simulink model "model_regulator"  (R2018a)
settings: Solver=ode45  StartTime=0.0  StopTime=500  RelTol=1e-3  EnableMultiTasking=on
values from neighbouring files (symbols this model uses):
  A = ans.A    [main.m]
  B = ans.B    [main.m]
  g1 = g(1)    [main.m]
  g2 = g(2)    [main.m]
  q11 = Q(1,1)    [main.m]
  q22 = Q(2,2)    [main.m]
  R = backup.R    [main.m]
undefined symbols (not defined in the file or in its folder): magnitude
libraries: simulink x3
settings Model: Creator=Vlad2  LastModifiedBy=Admin
settings DataIOCC: LimitDataPoints=on  SaveFormat=Array
settings OptimizationCC: LifeSpan=inf
settings DebuggingCC: SolverPrmCheckMsg=warning  SFUnexpectedBacktrackingDiag=warning  SFNoUnconditionalDefaultTransitionDiag=warning  SFExecutionAtInitializationDiag=none
settings HardwareCC: ProdBitPerPointer=32  ProdBitPerSizeT=32  ProdBitPerPtrDiffT=32  ProdLargestAtomicFloat=None  ProdIntDivRoundTo=Undefined  ProdEndianess=Unspecified  ProdWordSize=32  ProdHWDeviceType=32-bit Generic
settings ModelReferenceCC: PropagateSignalLabelsOutOfModel=off
settings CodeAppCC: StateflowObjectComments=on
settings GRTTargetCC: TargetLangStandard=C89/C90 (ANSI)  GeneratePreprocessorConditionals=Disable all
settings ConfigComp: CovMetricSettings=dw  CovHtmlReporting=on  CovSaveCumulativeToWorkspaceVar=on  CovSaveSingleToWorkspaceVar=on  CovExternalEMLEnable=off  CovSFcnEnable=off

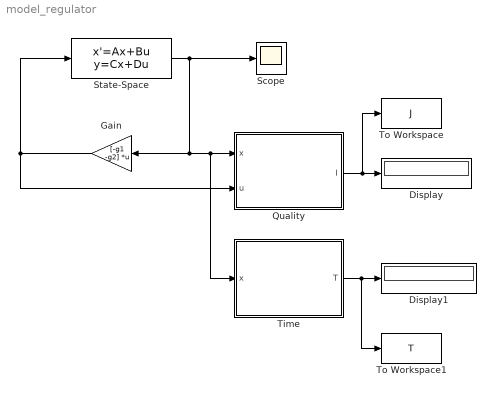
== system model_regulator ==
  Display : Display
  Display1 : Display
  Gain : Gain  Gain=[-g1 -g2]  Multiplication=Matrix(K*u)
  Quality : Subsystem
  Scope : Scope
  State-Space : StateSpace  A=A  B=B  C=eye(2)  D=[0;0]  InitialCondition=[1;1]
  "Time " : Subsystem
  To Workspace : ToWorkspace  VariableName=J  SaveFormat=Timeseries  SampleTime=-1
  To Workspace1 : ToWorkspace  VariableName=T  SaveFormat=Timeseries  SampleTime=-1
  wires:
  Quality/1(I) -> To Workspace/1, Display/1
  "Time "/1(T) -> To Workspace1/1, Display1/1
  Gain/1 -> Quality/2(u), State-Space/1
  State-Space/1 -> Scope/1, Gain/1, "Time "/1(x), Quality/1(x)

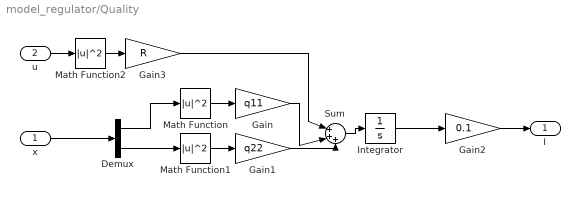
== system model_regulator/Quality ==
  x : Inport
  u : Inport  Port=2
  Demux : Demux  Outputs=2
  Gain : Gain  Gain=q11
  Gain1 : Gain  Gain=q22
  Gain2 : Gain  Gain=0.1
  Gain3 : Gain  Gain=R
  Integrator : Integrator
  Math Function : Math  Operator=magnitude^2  SaturateOnIntegerOverflow=on
  Math Function1 : Math  Operator=magnitude^2  SaturateOnIntegerOverflow=on
  Math Function2 : Math  Operator=magnitude^2  SaturateOnIntegerOverflow=on
  Sum : Sum  Inputs=|+++
  I : Outport
  wires:
  x/1 -> Demux/1
  Demux/1 -> Math Function/1
  Demux/2 -> Math Function1/1
  Math Function/1 -> Gain/1
  Math Function1/1 -> Gain1/1
  Math Function2/1 -> Gain3/1
  u/1 -> Math Function2/1
  Gain3/1 -> Sum/1
  Gain/1 -> Sum/2
  Gain1/1 -> Sum/3
  Sum/1 -> Integrator/1
  Integrator/1 -> Gain2/1
  Gain2/1 -> I/1

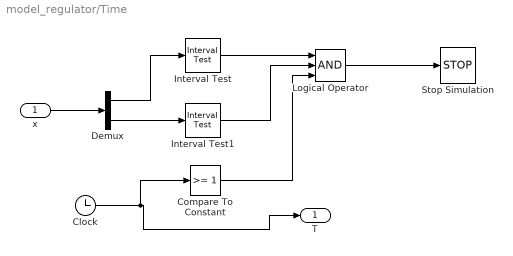
== system model_regulator/Time  ==
  x : Inport
  Clock : Clock
      settings: Decimation=10000
  Compare To Constant : simulink/Logic and Bit Operations/Compare To Constant  relop=>=  const=1  OutDataTypeStr=boolean
  Demux : Demux  Outputs=2
  Interval Test : simulink/Logic and Bit Operations/Interval Test  IntervalClosedRight=on  uplimit=0.001  IntervalClosedLeft=on  lowlimit=-0.001  OutDataTypeStr=boolean
  Interval Test1 : simulink/Logic and Bit Operations/Interval Test  IntervalClosedRight=on  uplimit=0.001  IntervalClosedLeft=on  lowlimit=-0.001  OutDataTypeStr=boolean
  Logical Operator : Logic  Inputs=3  AllPortsSameDT=off  OutDataTypeStr=boolean
  Stop Simulation : Stop
  T : Outport
  wires:
  x/1 -> Demux/1
  Logical Operator/1 -> Stop Simulation/1
  Demux/2 -> Interval Test1/1
  Demux/1 -> Interval Test/1
  Interval Test/1 -> Logical Operator/1
  Interval Test1/1 -> Logical Operator/2
  Compare To Constant/1 -> Logical Operator/3
  Clock/1 -> Compare To Constant/1, T/1
